simulink model "HL2"  (R2021b)
settings: Solver=FixedStepAuto  StartTime=0.0  StopTime=2  FixedStep=1/Fs  RelTol=1e-3
PreLoadFcn:
  | 50000
values from neighbouring files (symbols this model uses):
  Fs = 50000    [HL2.m]
libraries: fl_lib x208, ee_lib x58, nesl_utility x35
(part 1 of 3)
settings Model: Creator=fonzius  LastModifiedBy=fonzius

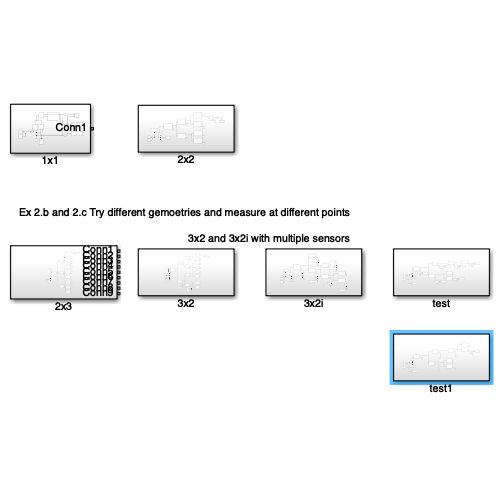
[thumbnail: Simulink's stored preview of the top-level diagram]
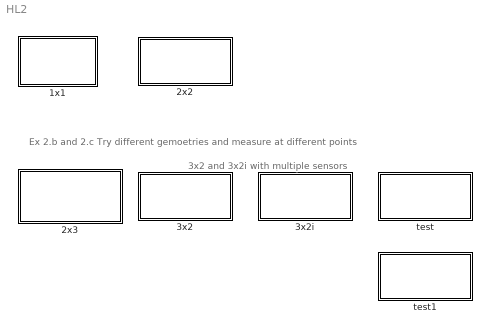
== system HL2 ==
  note: 3x2 and 3x2i with multiple sensors
  note: Ex 2.b and 2.c Try different gemoetries and measure at different points
  1x1 : Subsystem
  2x2 : Subsystem
  2x3 : Subsystem
  3x2 : Subsystem
  3x2i : Subsystem
  test : Subsystem
  test1 : Subsystem

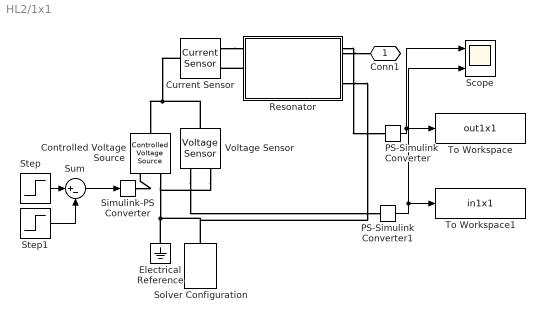
== system HL2/1x1 ==
  Controlled Voltage Source : fl_lib/Electrical/Electrical Sources/Controlled Voltage Source
  Current Sensor : fl_lib/Electrical/Electrical Sensors/Current Sensor
  Electrical Reference : fl_lib/Electrical/Electrical Elements/Electrical Reference
  PS-Simulink Converter : nesl_utility/PS-Simulink Converter  PhysicalDomain=network_engine_domain  SubClassName=ps_output  LeftPortType=input  RightPortType=output  PseudoPeriodic=off  Frequencies=[]  Unit=inherit  AffineConversion=off
      settings: SourceProductBaseCode=PW,SS
  PS-Simulink Converter1 : nesl_utility/PS-Simulink Converter  PhysicalDomain=network_engine_domain  SubClassName=ps_output  LeftPortType=input  RightPortType=output  PseudoPeriodic=off  Frequencies=[]  Unit=inherit  AffineConversion=off
      settings: SourceProductBaseCode=PW,SS
  Resonator : Subsystem
  Scope : Scope  NumInputPorts=2
  Simulink-PS Converter : nesl_utility/Simulink-PS Converter  PhysicalDomain=network_engine_domain  SubClassName=ps_input  LeftPortType=input  RightPortType=output  PseudoPeriodic=off  Frequencies=[]  NoiseDistribution=none  NoiseParameters=[]  Unit=1  AffineConversion=off  FilteringAndDerivatives=provide  SimscapeFilterOrder=1  InputFilterTimeConstant=0.001  UdotUserProvided=0
      settings: SourceProductBaseCode=PW,SS
  Solver Configuration : nesl_utility/Solver Configuration  PhysicalDomain=network_engine_domain  SubClassName=solver  LeftPortType=input  RightPortType=generic  Tones=[]  Harmonics=[]  SimulateNoise=off  Profile=off  UseLocalSampling=off  EnableSwitchedLinearOptims=on  FrequencyDomain=off  UseCCode=off  RelTol=0.001  AbsTol=1e-06  MinStep=1e-09  ToWorkspace=off  RevertToSquareIcSolve=off  NumHomotopyIterations=100  PhasorMode=off  PhasorModeNumHarmonics=1  DoDC=on  ResidualTolerance=1e-09  UseLocalSolver=off  LocalSolverChoice=NE_BACKWARD_EULER_ADVANCER  LocalSolverSampleTime=0.001  DoFixedCost=off  MaxNonlinIter=3  MaxModeIter=2  ComputeImpulses=off  ImpulseIterations=2  LinearAlgebra=auto  EquationFormulation=NE_TIME_EF  DelaysMemoryBudget=1024  AutomaticFiltering=on  FilteringTimeConstant=0.001  PartitionStorageMethod=AS_NEEDED  PartitionMemoryBudget=1024  PartitionMethod=ROBUST
      settings: SourceProductBaseCode=PW,SS
  Step : Step  Time=1/Fs  SampleTime=0
  Step1 : Step  Time=2/Fs  SampleTime=0
  Sum : Sum  Inputs=|+-
  To Workspace : ToWorkspace  VariableName=out1x1  SaveFormat=Timeseries  SampleTime=-1
  To Workspace1 : ToWorkspace  VariableName=in1x1  SaveFormat=Timeseries  SampleTime=-1
  Voltage Sensor : fl_lib/Electrical/Electrical Sensors/Voltage Sensor
  Conn1 : PMIOPort  Side=Right
  wires:
  Sum/1 -> Simulink-PS Converter/1
  PS-Simulink Converter/1 -> To Workspace/1, Scope/1
  Step/1 -> Sum/1
  PS-Simulink Converter1/1 -> Scope/2, To Workspace1/1
  Step1/1 -> Sum/2
  connections:
  Voltage Sensor/RConn1 -- PS-Simulink Converter1/LConn1
  Current Sensor/RConn1 -- PS-Simulink Converter/LConn1
  Electrical Reference/LConn1 -- Resonator/RConn2 -- Solver Configuration/RConn1 -- Voltage Sensor/RConn2 -- Controlled Voltage Source/RConn2
  Resonator/LConn1 -- Current Sensor/RConn2
  Simulink-PS Converter/RConn1 -- Controlled Voltage Source/RConn1
  Resonator/RConn1 -- Conn1/RConn1
  Voltage Sensor/LConn1 -- Current Sensor/LConn1 -- Controlled Voltage Source/LConn1

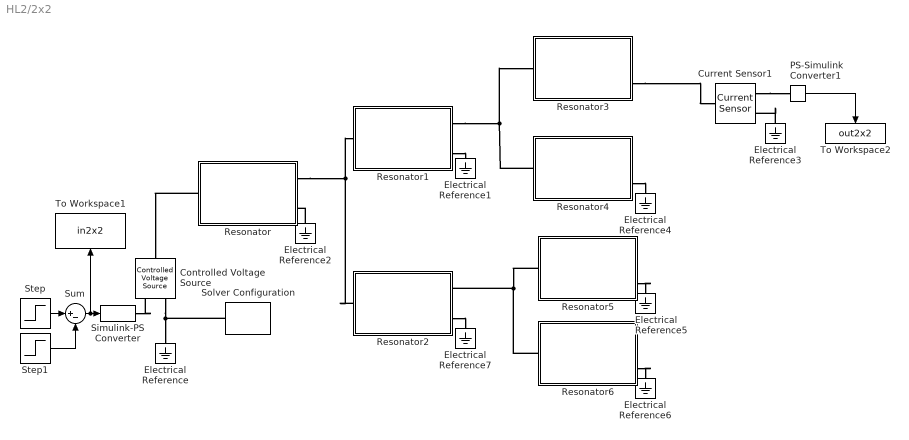
== system HL2/2x2 ==
  Controlled Voltage Source : fl_lib/Electrical/Electrical Sources/Controlled Voltage Source
  Current Sensor1 : fl_lib/Electrical/Electrical Sensors/Current Sensor
  Electrical Reference{,1..7} (8 alike) : fl_lib/Electrical/Electrical Elements/Electrical Reference
  PS-Simulink Converter1 : nesl_utility/PS-Simulink Converter  PhysicalDomain=network_engine_domain  SubClassName=ps_output  LeftPortType=input  RightPortType=output  PseudoPeriodic=off  Frequencies=[]  Unit=inherit  AffineConversion=off
      settings: SourceProductBaseCode=PW,SS
  Resonator : Subsystem
  Resonator1 : Subsystem
  Resonator2 : Subsystem
  Resonator3 : Subsystem
  Resonator4 : Subsystem
  Resonator5 : Subsystem
  Resonator6 : Subsystem
  Simulink-PS Converter : nesl_utility/Simulink-PS Converter  PhysicalDomain=network_engine_domain  SubClassName=ps_input  LeftPortType=input  RightPortType=output  PseudoPeriodic=off  Frequencies=[]  NoiseDistribution=none  NoiseParameters=[]  Unit=1  AffineConversion=off  FilteringAndDerivatives=provide  SimscapeFilterOrder=1  InputFilterTimeConstant=0.001  UdotUserProvided=0
      settings: SourceProductBaseCode=PW,SS
  Solver Configuration : nesl_utility/Solver Configuration  PhysicalDomain=network_engine_domain  SubClassName=solver  LeftPortType=input  RightPortType=generic  Tones=[]  Harmonics=[]  SimulateNoise=off  Profile=off  UseLocalSampling=off  EnableSwitchedLinearOptims=on  FrequencyDomain=off  UseCCode=off  RelTol=0.001  AbsTol=1e-06  MinStep=1e-09  ToWorkspace=off  RevertToSquareIcSolve=off  NumHomotopyIterations=100  PhasorMode=off  PhasorModeNumHarmonics=1  DoDC=on  ResidualTolerance=1e-09  UseLocalSolver=off  LocalSolverChoice=NE_BACKWARD_EULER_ADVANCER  LocalSolverSampleTime=0.001  DoFixedCost=off  MaxNonlinIter=3  MaxModeIter=2  ComputeImpulses=off  ImpulseIterations=2  LinearAlgebra=auto  EquationFormulation=NE_TIME_EF  DelaysMemoryBudget=1024  AutomaticFiltering=on  FilteringTimeConstant=0.001  PartitionStorageMethod=AS_NEEDED  PartitionMemoryBudget=1024  PartitionMethod=ROBUST
      settings: SourceProductBaseCode=PW,SS
  Step : Step  Time=1/Fs  SampleTime=0
  Step1 : Step  Time=2/Fs  SampleTime=0
  Sum : Sum  Inputs=|+-
  To Workspace1 : ToWorkspace  VariableName=in2x2  SaveFormat=Timeseries  SampleTime=-1
  To Workspace2 : ToWorkspace  VariableName=out2x2  SaveFormat=Timeseries  SampleTime=-1
  wires:
  Step1/1 -> Sum/2
  Step/1 -> Sum/1
  Sum/1 -> To Workspace1/1, Simulink-PS Converter/1
  PS-Simulink Converter1/1 -> To Workspace2/1
  connections:
  Resonator2/RConn2 -- Electrical Reference7/LConn1
  Resonator/RConn1 -- Resonator1/LConn1 -- Resonator2/LConn1
  Resonator5/RConn2 -- Electrical Reference5/LConn1
  Resonator4/RConn2 -- Electrical Reference4/LConn1
  Resonator1/RConn1 -- Resonator3/LConn1 -- Resonator4/LConn1
  Resonator5/LConn1 -- Resonator6/LConn1 -- Resonator2/RConn1
  Resonator6/RConn2 -- Electrical Reference6/LConn1
  Resonator/LConn1 -- Controlled Voltage Source/LConn1
  Simulink-PS Converter/RConn1 -- Controlled Voltage Source/RConn1
  Solver Configuration/RConn1 -- Electrical Reference/LConn1 -- Controlled Voltage Source/RConn2
  Current Sensor1/RConn1 -- PS-Simulink Converter1/LConn1
  Electrical Reference3/LConn1 -- Current Sensor1/RConn2
  Electrical Reference2/LConn1 -- Resonator/RConn2
  Resonator3/RConn2 -- Current Sensor1/LConn1
  Resonator1/RConn2 -- Electrical Reference1/LConn1

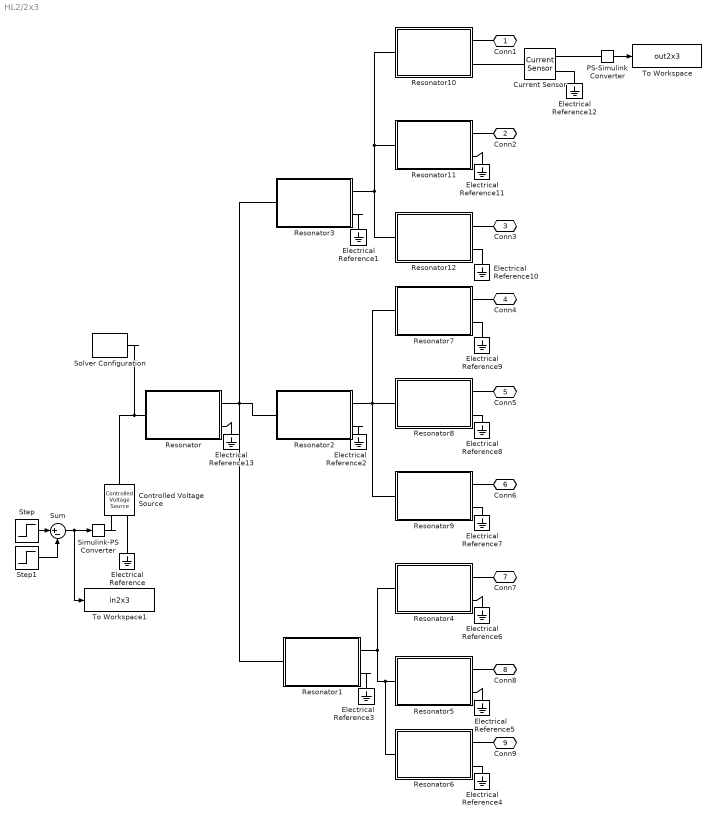
== system HL2/2x3 ==
  Controlled Voltage Source : fl_lib/Electrical/Electrical Sources/Controlled Voltage Source
  Current Sensor : fl_lib/Electrical/Electrical Sensors/Current Sensor
  Electrical Reference{,1..13} (14 alike) : fl_lib/Electrical/Electrical Elements/Electrical Reference
  PS-Simulink Converter : nesl_utility/PS-Simulink Converter  PhysicalDomain=network_engine_domain  SubClassName=ps_output  LeftPortType=input  RightPortType=output  PseudoPeriodic=off  Frequencies=[]  Unit=inherit  AffineConversion=off
      settings: SourceProductBaseCode=PW,SS
  Resonator : Subsystem
  Resonator1 : Subsystem
  Resonator10 : Subsystem
  Resonator11 : Subsystem
  Resonator12 : Subsystem
  Resonator2 : Subsystem
  Resonator3 : Subsystem
  Resonator4 : Subsystem
  Resonator5 : Subsystem
  Resonator6 : Subsystem
  Resonator7 : Subsystem
  Resonator8 : Subsystem
  Resonator9 : Subsystem
  Simulink-PS Converter : nesl_utility/Simulink-PS Converter  PhysicalDomain=network_engine_domain  SubClassName=ps_input  LeftPortType=input  RightPortType=output  PseudoPeriodic=off  Frequencies=[]  NoiseDistribution=none  NoiseParameters=[]  Unit=1  AffineConversion=off  FilteringAndDerivatives=provide  SimscapeFilterOrder=1  InputFilterTimeConstant=0.001  UdotUserProvided=0
      settings: SourceProductBaseCode=PW,SS
  Solver Configuration : nesl_utility/Solver Configuration  PhysicalDomain=network_engine_domain  SubClassName=solver  LeftPortType=input  RightPortType=generic  Tones=[]  Harmonics=[]  SimulateNoise=off  Profile=off  UseLocalSampling=off  EnableSwitchedLinearOptims=on  FrequencyDomain=off  UseCCode=off  RelTol=0.001  AbsTol=1e-06  MinStep=1e-09  ToWorkspace=off  RevertToSquareIcSolve=off  NumHomotopyIterations=100  PhasorMode=off  PhasorModeNumHarmonics=1  DoDC=on  ResidualTolerance=1e-09  UseLocalSolver=off  LocalSolverChoice=NE_BACKWARD_EULER_ADVANCER  LocalSolverSampleTime=0.001  DoFixedCost=off  MaxNonlinIter=3  MaxModeIter=2  ComputeImpulses=off  ImpulseIterations=2  LinearAlgebra=auto  EquationFormulation=NE_TIME_EF  DelaysMemoryBudget=1024  AutomaticFiltering=on  FilteringTimeConstant=0.001  PartitionStorageMethod=AS_NEEDED  PartitionMemoryBudget=1024  PartitionMethod=ROBUST
      settings: SourceProductBaseCode=PW,SS
  Step : Step  Time=1/Fs  SampleTime=0
  Step1 : Step  Time=2/Fs  SampleTime=0
  Sum : Sum  Inputs=|+-
  To Workspace : ToWorkspace  VariableName=out2x3  SaveFormat=Timeseries  SampleTime=-1
  To Workspace1 : ToWorkspace  VariableName=in2x3  SaveFormat=Timeseries  SampleTime=-1
  Conn1 : PMIOPort  Side=Right
  Conn2 : PMIOPort  Port=2  Side=Right
  Conn3 : PMIOPort  Port=3  Side=Right
  Conn4 : PMIOPort  Port=4  Side=Right
  Conn5 : PMIOPort  Port=5  Side=Right
  Conn6 : PMIOPort  Port=6  Side=Right
  Conn7 : PMIOPort  Port=7  Side=Right
  Conn8 : PMIOPort  Port=8  Side=Right
  Conn9 : PMIOPort  Port=9  Side=Right
  wires:
  Step/1 -> Sum/1
  Sum/1 -> To Workspace1/1, Simulink-PS Converter/1
  Step1/1 -> Sum/2
  PS-Simulink Converter/1 -> To Workspace/1
  connections:
  Resonator9/RConn1 -- Conn6/RConn1
  Resonator11/RConn1 -- Conn2/RConn1
  Resonator12/RConn1 -- Conn3/RConn1
  Resonator7/RConn2 -- Electrical Reference9/LConn1
  Resonator1/RConn2 -- Electrical Reference3/LConn1
  Resonator9/RConn2 -- Electrical Reference7/LConn1
  Resonator3/RConn2 -- Electrical Reference1/LConn1
  Resonator2/RConn2 -- Electrical Reference2/LConn1
  Simulink-PS Converter/RConn1 -- Controlled Voltage Source/RConn1
  Resonator6/RConn1 -- Conn9/RConn1
  Resonator4/RConn1 -- Conn7/RConn1
  Electrical Reference11/LConn1 -- Resonator11/RConn2
  Resonator4/LConn1 -- Resonator6/LConn1 -- Resonator5/LConn1 -- Resonator1/RConn1
  Resonator/RConn1 -- Resonator1/LConn1 -- Resonator3/LConn1 -- Resonator2/LConn1
  Electrical Reference5/LConn1 -- Resonator5/RConn2
  Resonator7/RConn1 -- Conn4/RConn1
  Resonator10/RConn2 -- Current Sensor/LConn1
  Solver Configuration/RConn1 -- Controlled Voltage Source/LConn1 -- Resonator/LConn1
  Resonator2/RConn1 -- Resonator8/LConn1 -- Resonator9/LConn1 -- Resonator7/LConn1
  Resonator8/RConn1 -- Conn5/RConn1
  Resonator8/RConn2 -- Electrical Reference8/LConn1
  Resonator10/LConn1 -- Resonator11/LConn1 -- Resonator12/LConn1 -- Resonator3/RConn1
  Resonator12/RConn2 -- Electrical Reference10/LConn1
  Resonator10/RConn1 -- Conn1/RConn1
  Resonator6/RConn2 -- Electrical Reference4/LConn1
  Electrical Reference13/LConn1 -- Resonator/RConn2
  Resonator5/RConn1 -- Conn8/RConn1
  Electrical Reference6/LConn1 -- Resonator4/RConn2
  Controlled Voltage Source/RConn2 -- Electrical Reference/LConn1
  Current Sensor/RConn1 -- PS-Simulink Converter/LConn1
  Electrical Reference12/LConn1 -- Current Sensor/RConn2

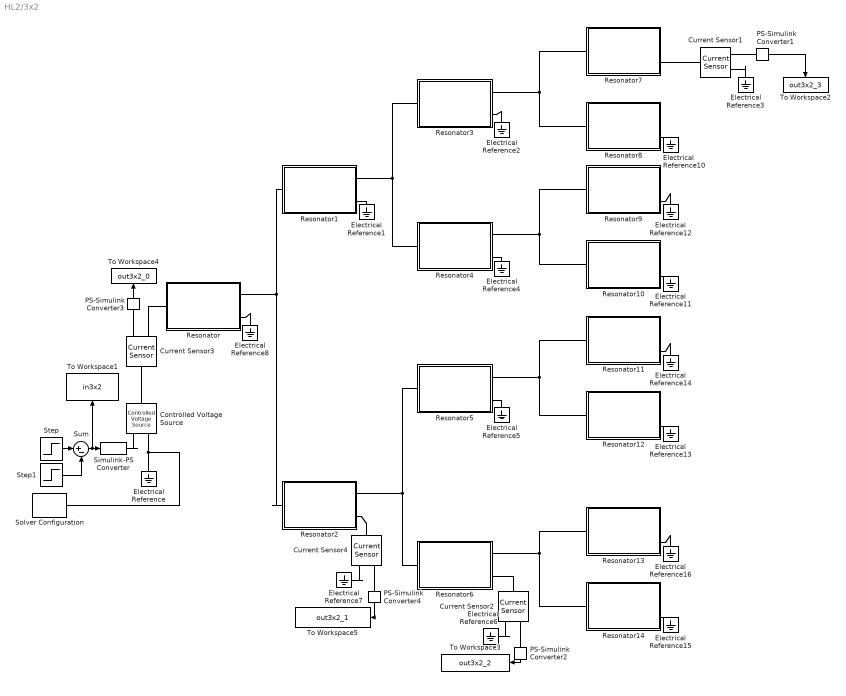
== system HL2/3x2 ==
  Controlled Voltage Source : fl_lib/Electrical/Electrical Sources/Controlled Voltage Source
  Current Sensor{1..4} (4 alike) : fl_lib/Electrical/Electrical Sensors/Current Sensor
  Electrical Reference{,1..8,10..16} (16 alike) : fl_lib/Electrical/Electrical Elements/Electrical Reference
  PS-Simulink Converter{1..4} (4 alike) : nesl_utility/PS-Simulink Converter  PhysicalDomain=network_engine_domain  SubClassName=ps_output  LeftPortType=input  RightPortType=output  PseudoPeriodic=off  Frequencies=[]  Unit=inherit  AffineConversion=off
      settings: SourceProductBaseCode=PW,SS
  Resonator : Subsystem
  Resonator1 : Subsystem
  Resonator10 : Subsystem
  Resonator11 : Subsystem
  Resonator12 : Subsystem
  Resonator13 : Subsystem
  Resonator14 : Subsystem
  Resonator2 : Subsystem
  Resonator3 : Subsystem
  Resonator4 : Subsystem
  Resonator5 : Subsystem
  Resonator6 : Subsystem
  Resonator7 : Subsystem
  Resonator8 : Subsystem
  Resonator9 : Subsystem
  Simulink-PS Converter : nesl_utility/Simulink-PS Converter  PhysicalDomain=network_engine_domain  SubClassName=ps_input  LeftPortType=input  RightPortType=output  PseudoPeriodic=off  Frequencies=[]  NoiseDistribution=none  NoiseParameters=[]  Unit=1  AffineConversion=off  FilteringAndDerivatives=provide  SimscapeFilterOrder=1  InputFilterTimeConstant=0.001  UdotUserProvided=0
      settings: SourceProductBaseCode=PW,SS
  Solver Configuration : nesl_utility/Solver Configuration  PhysicalDomain=network_engine_domain  SubClassName=solver  LeftPortType=input  RightPortType=generic  Tones=[]  Harmonics=[]  SimulateNoise=off  Profile=off  UseLocalSampling=off  EnableSwitchedLinearOptims=on  FrequencyDomain=off  UseCCode=off  RelTol=0.001  AbsTol=1e-06  MinStep=1e-09  ToWorkspace=off  RevertToSquareIcSolve=off  NumHomotopyIterations=100  PhasorMode=off  PhasorModeNumHarmonics=1  DoDC=on  ResidualTolerance=1e-09  UseLocalSolver=off  LocalSolverChoice=NE_BACKWARD_EULER_ADVANCER  LocalSolverSampleTime=0.001  DoFixedCost=off  MaxNonlinIter=3  MaxModeIter=2  ComputeImpulses=off  ImpulseIterations=2  LinearAlgebra=auto  EquationFormulation=NE_TIME_EF  DelaysMemoryBudget=1024  AutomaticFiltering=on  FilteringTimeConstant=0.001  PartitionStorageMethod=AS_NEEDED  PartitionMemoryBudget=1024  PartitionMethod=ROBUST
      settings: SourceProductBaseCode=PW,SS
  Step : Step  Time=1/Fs  SampleTime=0
  Step1 : Step  Time=2/Fs  SampleTime=0
  Sum : Sum  Inputs=|+-
  To Workspace1 : ToWorkspace  VariableName=in3x2  SaveFormat=Timeseries  SampleTime=-1
  To Workspace2 : ToWorkspace  VariableName=out3x2_3  SaveFormat=Timeseries  SampleTime=-1
  To Workspace3 : ToWorkspace  VariableName=out3x2_2  SaveFormat=Timeseries  SampleTime=-1
  To Workspace4 : ToWorkspace  VariableName=out3x2_0  SaveFormat=Timeseries  SampleTime=-1
  To Workspace5 : ToWorkspace  VariableName=out3x2_1  SaveFormat=Timeseries  SampleTime=-1
  wires:
  Step1/1 -> Sum/2
  Step/1 -> Sum/1
  Sum/1 -> To Workspace1/1, Simulink-PS Converter/1
  PS-Simulink Converter3/1 -> To Workspace4/1
  PS-Simulink Converter1/1 -> To Workspace2/1
  PS-Simulink Converter2/1 -> To Workspace3/1
  PS-Simulink Converter4/1 -> To Workspace5/1
  connections:
  Current Sensor4/LConn1 -- Resonator2/RConn2
  Resonator/RConn1 -- Resonator1/LConn1 -- Resonator2/LConn1
  Resonator5/RConn2 -- Electrical Reference5/LConn1
  Resonator4/RConn2 -- Electrical Reference4/LConn1
  Resonator1/RConn1 -- Resonator4/LConn1 -- Resonator3/LConn1
  Resonator5/LConn1 -- Resonator6/LConn1 -- Resonator2/RConn1
  Current Sensor2/LConn1 -- Resonator6/RConn2
  Simulink-PS Converter/RConn1 -- Controlled Voltage Source/RConn1
  Solver Configuration/RConn1 -- Electrical Reference/LConn1 -- Controlled Voltage Source/RConn2
  Current Sensor3/RConn1 -- PS-Simulink Converter3/LConn1
  Resonator1/RConn2 -- Electrical Reference1/LConn1
  Electrical Reference3/LConn1 -- Current Sensor1/RConn2
  Current Sensor1/RConn1 -- PS-Simulink Converter1/LConn1
  Electrical Reference2/LConn1 -- Resonator3/RConn2
  Resonator8/RConn2 -- Electrical Reference10/LConn1
  Resonator7/RConn2 -- Current Sensor1/LConn1
  Resonator7/LConn1 -- Resonator8/LConn1 -- Resonator3/RConn1
  Electrical Reference12/LConn1 -- Resonator9/RConn2
  Resonator10/RConn2 -- Electrical Reference11/LConn1
  Resonator9/LConn1 -- Resonator10/LConn1 -- Resonator4/RConn1
  Electrical Reference14/LConn1 -- Resonator11/RConn2
  Resonator12/RConn2 -- Electrical Reference13/LConn1
  Resonator11/LConn1 -- Resonator12/LConn1 -- Resonator5/RConn1
  Electrical Reference16/LConn1 -- Resonator13/RConn2
  Resonator14/RConn2 -- Electrical Reference15/LConn1
  Resonator6/RConn1 -- Resonator14/LConn1 -- Resonator13/LConn1
  Electrical Reference8/LConn1 -- Resonator/RConn2
  Current Sensor3/LConn1 -- Controlled Voltage Source/LConn1
  Resonator/LConn1 -- Current Sensor3/RConn2
  Current Sensor2/RConn1 -- PS-Simulink Converter2/LConn1
  Electrical Reference6/LConn1 -- Current Sensor2/RConn2
  Electrical Reference7/LConn1 -- Current Sensor4/RConn2
  Current Sensor4/RConn1 -- PS-Simulink Converter4/LConn1

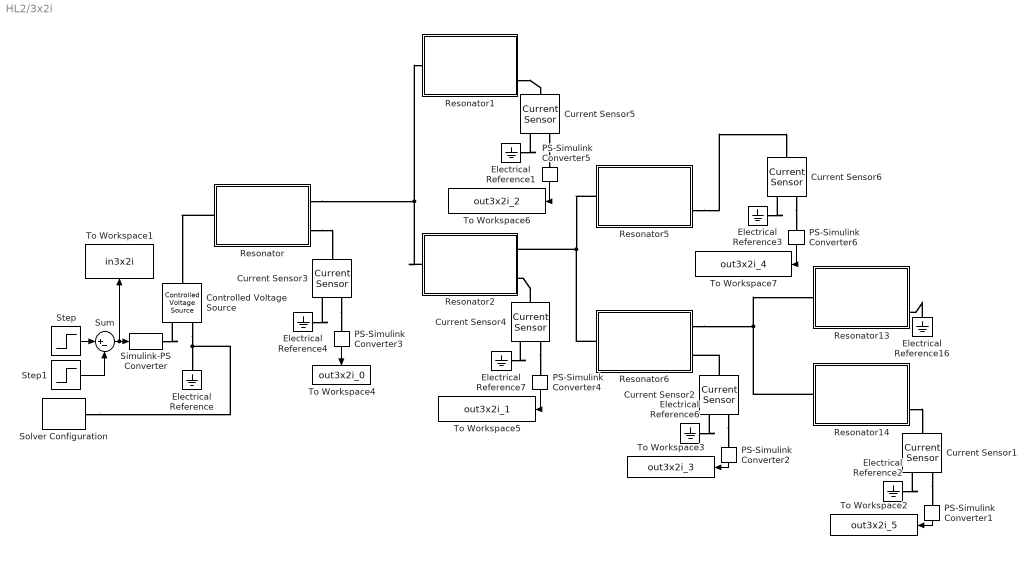
== system HL2/3x2i ==
  Controlled Voltage Source : fl_lib/Electrical/Electrical Sources/Controlled Voltage Source
  Current Sensor{1..6} (6 alike) : fl_lib/Electrical/Electrical Sensors/Current Sensor
  Electrical Reference{,1..4,6..7,16} (8 alike) : fl_lib/Electrical/Electrical Elements/Electrical Reference
  PS-Simulink Converter{1..6} (6 alike) : nesl_utility/PS-Simulink Converter  PhysicalDomain=network_engine_domain  SubClassName=ps_output  LeftPortType=input  RightPortType=output  PseudoPeriodic=off  Frequencies=[]  Unit=inherit  AffineConversion=off
      settings: SourceProductBaseCode=PW,SS
  Resonator : Subsystem
  Resonator1 : Subsystem
  Resonator13 : Subsystem
  Resonator14 : Subsystem
  Resonator2 : Subsystem
  Resonator5 : Subsystem
  Resonator6 : Subsystem
  Simulink-PS Converter : nesl_utility/Simulink-PS Converter  PhysicalDomain=network_engine_domain  SubClassName=ps_input  LeftPortType=input  RightPortType=output  PseudoPeriodic=off  Frequencies=[]  NoiseDistribution=none  NoiseParameters=[]  Unit=1  AffineConversion=off  FilteringAndDerivatives=provide  SimscapeFilterOrder=1  InputFilterTimeConstant=0.001  UdotUserProvided=0
      settings: SourceProductBaseCode=PW,SS
  Solver Configuration : nesl_utility/Solver Configuration  PhysicalDomain=network_engine_domain  SubClassName=solver  LeftPortType=input  RightPortType=generic  Tones=[]  Harmonics=[]  SimulateNoise=off  Profile=off  UseLocalSampling=off  EnableSwitchedLinearOptims=on  FrequencyDomain=off  UseCCode=off  RelTol=0.001  AbsTol=1e-06  MinStep=1e-09  ToWorkspace=off  RevertToSquareIcSolve=off  NumHomotopyIterations=100  PhasorMode=off  PhasorModeNumHarmonics=1  DoDC=on  ResidualTolerance=1e-09  UseLocalSolver=off  LocalSolverChoice=NE_BACKWARD_EULER_ADVANCER  LocalSolverSampleTime=0.001  DoFixedCost=off  MaxNonlinIter=3  MaxModeIter=2  ComputeImpulses=off  ImpulseIterations=2  LinearAlgebra=auto  EquationFormulation=NE_TIME_EF  DelaysMemoryBudget=1024  AutomaticFiltering=on  FilteringTimeConstant=0.001  PartitionStorageMethod=AS_NEEDED  PartitionMemoryBudget=1024  PartitionMethod=ROBUST
      settings: SourceProductBaseCode=PW,SS
  Step : Step  Time=1/Fs  SampleTime=0
  Step1 : Step  Time=2/Fs  SampleTime=0
  Sum : Sum  Inputs=|+-
  To Workspace1 : ToWorkspace  VariableName=in3x2i  SaveFormat=Timeseries  SampleTime=-1
  To Workspace2 : ToWorkspace  VariableName=out3x2i_5  SaveFormat=Timeseries  SampleTime=-1
  To Workspace3 : ToWorkspace  VariableName=out3x2i_3  SaveFormat=Timeseries  SampleTime=-1
  To Workspace4 : ToWorkspace  VariableName=out3x2i_0  SaveFormat=Timeseries  SampleTime=-1
  To Workspace5 : ToWorkspace  VariableName=out3x2i_1  SaveFormat=Timeseries  SampleTime=-1
  To Workspace6 : ToWorkspace  VariableName=out3x2i_2  SaveFormat=Timeseries  SampleTime=-1
  To Workspace7 : ToWorkspace  VariableName=out3x2i_4  SaveFormat=Timeseries  SampleTime=-1
  wires:
  Step1/1 -> Sum/2
  Step/1 -> Sum/1
  Sum/1 -> To Workspace1/1, Simulink-PS Converter/1
  PS-Simulink Converter2/1 -> To Workspace3/1
  PS-Simulink Converter4/1 -> To Workspace5/1
  PS-Simulink Converter1/1 -> To Workspace2/1
  PS-Simulink Converter5/1 -> To Workspace6/1
  PS-Simulink Converter6/1 -> To Workspace7/1
  PS-Simulink Converter3/1 -> To Workspace4/1
  connections:
  Current Sensor4/LConn1 -- Resonator2/RConn2
  Resonator/RConn1 -- Resonator1/LConn1 -- Resonator2/LConn1
  Resonator5/RConn2 -- Current Sensor6/LConn1
  Resonator5/LConn1 -- Resonator6/LConn1 -- Resonator2/RConn1
  Current Sensor2/LConn1 -- Resonator6/RConn2
  Simulink-PS Converter/RConn1 -- Controlled Voltage Source/RConn1
  Solver Configuration/RConn1 -- Electrical Reference/LConn1 -- Controlled Voltage Source/RConn2
  Resonator1/RConn2 -- Current Sensor5/LConn1
  Electrical Reference16/LConn1 -- Resonator13/RConn2
  Resonator14/RConn2 -- Current Sensor1/LConn1
  Resonator6/RConn1 -- Resonator13/LConn1 -- Resonator14/LConn1
  Resonator/LConn1 -- Controlled Voltage Source/LConn1
  Current Sensor2/RConn1 -- PS-Simulink Converter2/LConn1
  Electrical Reference6/LConn1 -- Current Sensor2/RConn2
  Electrical Reference7/LConn1 -- Current Sensor4/RConn2
  Current Sensor4/RConn1 -- PS-Simulink Converter4/LConn1
  Current Sensor1/RConn1 -- PS-Simulink Converter1/LConn1
  Electrical Reference2/LConn1 -- Current Sensor1/RConn2
  Electrical Reference1/LConn1 -- Current Sensor5/RConn2
  Current Sensor5/RConn1 -- PS-Simulink Converter5/LConn1
  Electrical Reference3/LConn1 -- Current Sensor6/RConn2
  Current Sensor6/RConn1 -- PS-Simulink Converter6/LConn1
  Current Sensor3/RConn1 -- PS-Simulink Converter3/LConn1
  Electrical Reference4/LConn1 -- Current Sensor3/RConn2
  Resonator/RConn2 -- Current Sensor3/LConn1

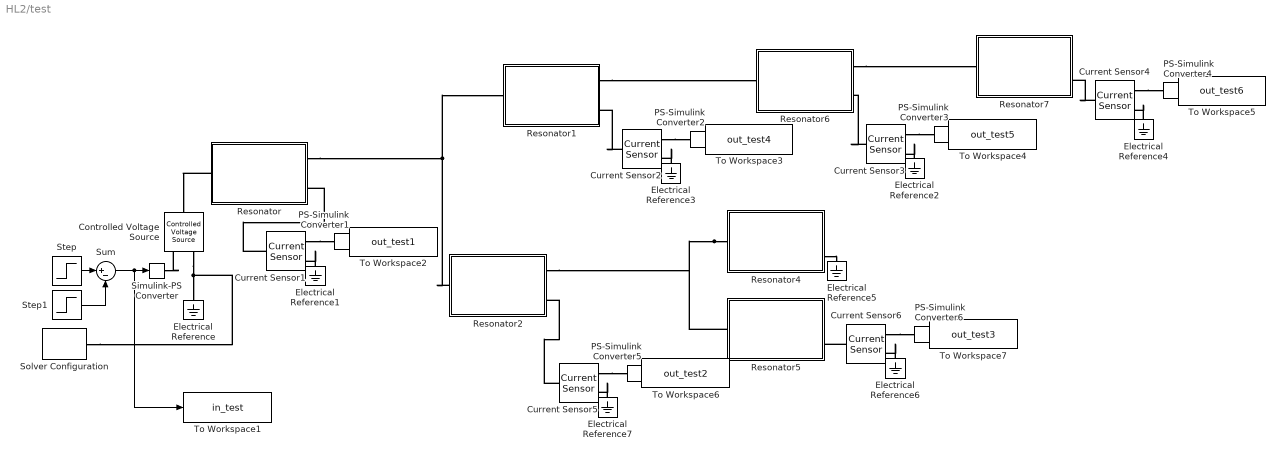
== system HL2/test ==
  Controlled Voltage Source : fl_lib/Electrical/Electrical Sources/Controlled Voltage Source
  Current Sensor{1..6} (6 alike) : fl_lib/Electrical/Electrical Sensors/Current Sensor
  Electrical Reference{,1..7} (8 alike) : fl_lib/Electrical/Electrical Elements/Electrical Reference
  PS-Simulink Converter{1..6} (6 alike) : nesl_utility/PS-Simulink Converter  PhysicalDomain=network_engine_domain  SubClassName=ps_output  LeftPortType=input  RightPortType=output  PseudoPeriodic=off  Frequencies=[]  Unit=inherit  AffineConversion=off
      settings: SourceProductBaseCode=PW,SS
  Resonator : Subsystem
  Resonator1 : Subsystem
  Resonator2 : Subsystem
  Resonator4 : Subsystem
  Resonator5 : Subsystem
  Resonator6 : Subsystem
  Resonator7 : Subsystem
  Simulink-PS Converter : nesl_utility/Simulink-PS Converter  PhysicalDomain=network_engine_domain  SubClassName=ps_input  LeftPortType=input  RightPortType=output  PseudoPeriodic=off  Frequencies=[]  NoiseDistribution=none  NoiseParameters=[]  Unit=1  AffineConversion=off  FilteringAndDerivatives=provide  SimscapeFilterOrder=1  InputFilterTimeConstant=0.001  UdotUserProvided=0
      settings: SourceProductBaseCode=PW,SS
  Solver Configuration : nesl_utility/Solver Configuration  PhysicalDomain=network_engine_domain  SubClassName=solver  LeftPortType=input  RightPortType=generic  Tones=[]  Harmonics=[]  SimulateNoise=off  Profile=off  UseLocalSampling=off  EnableSwitchedLinearOptims=on  FrequencyDomain=off  UseCCode=off  RelTol=0.001  AbsTol=1e-06  MinStep=1e-09  ToWorkspace=off  RevertToSquareIcSolve=off  NumHomotopyIterations=100  PhasorMode=off  PhasorModeNumHarmonics=1  DoDC=on  ResidualTolerance=1e-09  UseLocalSolver=off  LocalSolverChoice=NE_BACKWARD_EULER_ADVANCER  LocalSolverSampleTime=0.001  DoFixedCost=off  MaxNonlinIter=3  MaxModeIter=2  ComputeImpulses=off  ImpulseIterations=2  LinearAlgebra=auto  EquationFormulation=NE_TIME_EF  DelaysMemoryBudget=1024  AutomaticFiltering=on  FilteringTimeConstant=0.001  PartitionStorageMethod=AS_NEEDED  PartitionMemoryBudget=1024  PartitionMethod=ROBUST
      settings: SourceProductBaseCode=PW,SS
  Step : Step  Time=1/Fs  SampleTime=0
  Step1 : Step  Time=2/Fs  SampleTime=0
  Sum : Sum  Inputs=|+-
  To Workspace1 : ToWorkspace  VariableName=in_test  SaveFormat=Timeseries  SampleTime=-1
  To Workspace2 : ToWorkspace  VariableName=out_test1  SaveFormat=Timeseries  SampleTime=-1
  To Workspace3 : ToWorkspace  VariableName=out_test4  SaveFormat=Timeseries  SampleTime=-1
  To Workspace4 : ToWorkspace  VariableName=out_test5  SaveFormat=Timeseries  SampleTime=-1
  To Workspace5 : ToWorkspace  VariableName=out_test6  SaveFormat=Timeseries  SampleTime=-1
  To Workspace6 : ToWorkspace  VariableName=out_test2  SaveFormat=Timeseries  SampleTime=-1
  To Workspace7 : ToWorkspace  VariableName=out_test3  SaveFormat=Timeseries  SampleTime=-1
  wires:
  Step/1 -> Sum/1
  Step1/1 -> Sum/2
  Sum/1 -> To Workspace1/1, Simulink-PS Converter/1
  PS-Simulink Converter2/1 -> To Workspace3/1
  PS-Simulink Converter3/1 -> To Workspace4/1
  PS-Simulink Converter4/1 -> To Workspace5/1
  PS-Simulink Converter5/1 -> To Workspace6/1
  PS-Simulink Converter6/1 -> To Workspace7/1
  PS-Simulink Converter1/1 -> To Workspace2/1
  connections:
  Resonator2/LConn1 -- Resonator/RConn1 -- Resonator1/LConn1
  Resonator4/LConn1 -- Resonator2/RConn1 -- Resonator5/LConn1
  Controlled Voltage Source/RConn2 -- Solver Configuration/RConn1 -- Electrical Reference/LConn1
  Current Sensor6/LConn1 -- Resonator5/RConn2
  Current Sensor3/LConn1 -- Resonator6/RConn2
  Resonator/LConn1 -- Controlled Voltage Source/LConn1
  Current Sensor5/LConn1 -- Resonator2/RConn2
  Current Sensor2/LConn1 -- Resonator1/RConn2
  Resonator4/RConn2 -- Electrical Reference5/LConn1
  Current Sensor4/LConn1 -- Resonator7/RConn2
  Simulink-PS Converter/RConn1 -- Controlled Voltage Source/RConn1
  Resonator1/RConn1 -- Resonator6/LConn1
  Resonator6/RConn1 -- Resonator7/LConn1
  Electrical Reference3/LConn1 -- Current Sensor2/RConn2
  Current Sensor2/RConn1 -- PS-Simulink Converter2/LConn1
  Electrical Reference2/LConn1 -- Current Sensor3/RConn2
  Current Sensor3/RConn1 -- PS-Simulink Converter3/LConn1
  Electrical Reference4/LConn1 -- Current Sensor4/RConn2
  Current Sensor4/RConn1 -- PS-Simulink Converter4/LConn1
  Electrical Reference7/LConn1 -- Current Sensor5/RConn2
  Current Sensor5/RConn1 -- PS-Simulink Converter5/LConn1
  Electrical Reference6/LConn1 -- Current Sensor6/RConn2
  Current Sensor6/RConn1 -- PS-Simulink Converter6/LConn1
  Electrical Reference1/LConn1 -- Current Sensor1/RConn2
  Current Sensor1/RConn1 -- PS-Simulink Converter1/LConn1
  Current Sensor1/LConn1 -- Resonator/RConn2

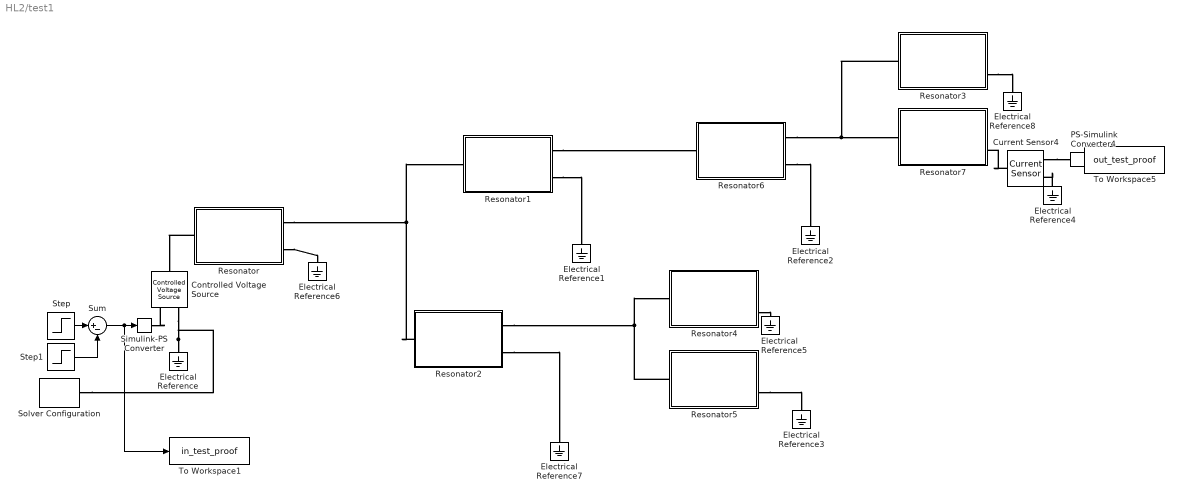
== system HL2/test1 ==
  Controlled Voltage Source : fl_lib/Electrical/Electrical Sources/Controlled Voltage Source
  Current Sensor4 : fl_lib/Electrical/Electrical Sensors/Current Sensor
  Electrical Reference{,1..8} (9 alike) : fl_lib/Electrical/Electrical Elements/Electrical Reference
  PS-Simulink Converter4 : nesl_utility/PS-Simulink Converter  PhysicalDomain=network_engine_domain  SubClassName=ps_output  LeftPortType=input  RightPortType=output  PseudoPeriodic=off  Frequencies=[]  Unit=inherit  AffineConversion=off
      settings: SourceProductBaseCode=PW,SS
  Resonator : Subsystem
  Resonator1 : Subsystem
  Resonator2 : Subsystem
  Resonator3 : Subsystem
  Resonator4 : Subsystem
  Resonator5 : Subsystem
  Resonator6 : Subsystem
  Resonator7 : Subsystem
  Simulink-PS Converter : nesl_utility/Simulink-PS Converter  PhysicalDomain=network_engine_domain  SubClassName=ps_input  LeftPortType=input  RightPortType=output  PseudoPeriodic=off  Frequencies=[]  NoiseDistribution=none  NoiseParameters=[]  Unit=1  AffineConversion=off  FilteringAndDerivatives=provide  SimscapeFilterOrder=1  InputFilterTimeConstant=0.001  UdotUserProvided=0
      settings: SourceProductBaseCode=PW,SS
  Solver Configuration : nesl_utility/Solver Configuration  PhysicalDomain=network_engine_domain  SubClassName=solver  LeftPortType=input  RightPortType=generic  Tones=[]  Harmonics=[]  SimulateNoise=off  Profile=off  UseLocalSampling=off  EnableSwitchedLinearOptims=on  FrequencyDomain=off  UseCCode=off  RelTol=0.001  AbsTol=1e-06  MinStep=1e-09  ToWorkspace=off  RevertToSquareIcSolve=off  NumHomotopyIterations=100  PhasorMode=off  PhasorModeNumHarmonics=1  DoDC=on  ResidualTolerance=1e-09  UseLocalSolver=off  LocalSolverChoice=NE_BACKWARD_EULER_ADVANCER  LocalSolverSampleTime=0.001  DoFixedCost=off  MaxNonlinIter=3  MaxModeIter=2  ComputeImpulses=off  ImpulseIterations=2  LinearAlgebra=auto  EquationFormulation=NE_TIME_EF  DelaysMemoryBudget=1024  AutomaticFiltering=on  FilteringTimeConstant=0.001  PartitionStorageMethod=AS_NEEDED  PartitionMemoryBudget=1024  PartitionMethod=ROBUST
      settings: SourceProductBaseCode=PW,SS
  Step : Step  Time=1/Fs  SampleTime=0
  Step1 : Step  Time=2/Fs  SampleTime=0
  Sum : Sum  Inputs=|+-
  To Workspace1 : ToWorkspace  VariableName=in_test_proof  SaveFormat=Timeseries  SampleTime=-1
  To Workspace5 : ToWorkspace  VariableName=out_test_proof  SaveFormat=Timeseries  SampleTime=-1
  wires:
  Step/1 -> Sum/1
  Step1/1 -> Sum/2
  Sum/1 -> To Workspace1/1, Simulink-PS Converter/1
  PS-Simulink Converter4/1 -> To Workspace5/1
  connections:
  Resonator2/LConn1 -- Resonator1/LConn1 -- Resonator/RConn1
  Resonator5/LConn1 -- Resonator4/LConn1 -- Resonator2/RConn1
  Electrical Reference/LConn1 -- Controlled Voltage Source/RConn2 -- Solver Configuration/RConn1
  Resonator5/RConn2 -- Electrical Reference3/LConn1
  Resonator6/RConn2 -- Electrical Reference2/LConn1
  Resonator/LConn1 -- Controlled Voltage Source/LConn1
  Resonator1/RConn2 -- Electrical Reference1/LConn1
  Resonator4/RConn2 -- Electrical Reference5/LConn1
  Current Sensor4/LConn1 -- Resonator7/RConn2
  Simulink-PS Converter/RConn1 -- Controlled Voltage Source/RConn1
  Resonator1/RConn1 -- Resonator6/LConn1
  Resonator6/RConn1 -- Resonator3/LConn1 -- Resonator7/LConn1
  Electrical Reference4/LConn1 -- Current Sensor4/RConn2
  Current Sensor4/RConn1 -- PS-Simulink Converter4/LConn1
  Resonator2/RConn2 -- Electrical Reference7/LConn1
  Resonator/RConn2 -- Electrical Reference6/LConn1
  Resonator3/RConn2 -- Electrical Reference8/LConn1

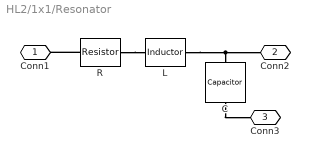
== system HL2/1x1/Resonator ==
  C : fl_lib/Electrical/Electrical Elements/Capacitor  c=7.0832e-07 F  r=0 Ohm  g=0 1/Ohm  i_specify=off  i_priority=None  i=0 A  i_nominal_specify=off  i_nominal_unit=A  i_nominal_value=1  v_specify=off  v_priority=None  v=0 V  v_nominal_specify=off  v_nominal_unit=V  v_nominal_value=1  vc_specify=off  vc_priority=High  vc=0 V  vc_nominal_specify=off  vc_nominal_unit=V  vc_nominal_value=1
  L : ee_lib/Passive/Inductor  l=0.10005 H  L_tol=0  enable_L_tol=0  tol_distribution=1  nSigma=4  r=0 Ohm  g=0 1/Ohm  enable_operating_limits=0  operating_limit_action=2  max_working_current=1 A  power_rating=1 W  enable_faults=0  fault_action=1  lambdaPercent=50  k_faulted=0.9999  turnsShort=0  openCct=0  groundShort=0  groundShortG=0 1/Ohm  tau_fault=1e-3 s  enable_temporal_fault=0  t_fault=1 s  enable_behavioral_fault=0  max_permissible_voltage=100 V  n_fail_on_voltage=1  max_permissible_current=1 A  t_fail_on_current=1 s  i_L_specify=off  i_L_priority=High  i_L=0 A  i_L_nominal_specify=off  i_L_nominal_unit=A  i_L_nominal_value=1
  R : fl_lib/Electrical/Electrical Elements/Resistor  R=4.116 Ohm  i_specify=off  i_priority=None  i=0 A  i_nominal_specify=off  i_nominal_unit=A  i_nominal_value=1  v_specify=off  v_priority=None  v=0 V  v_nominal_specify=off  v_nominal_unit=V  v_nominal_value=1
  Conn1 : PMIOPort  Side=Left
  Conn2 : PMIOPort  Port=2  Side=Right
  Conn3 : PMIOPort  Port=3  Side=Right
  connections:
  R/RConn1 -- L/LConn1
  C/RConn1 -- Conn3/RConn1
  R/LConn1 -- Conn1/RConn1
  L/RConn1 -- Conn2/RConn1 -- C/LConn1

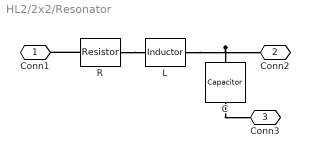
== system HL2/2x2/Resonator ==
  C : fl_lib/Electrical/Electrical Elements/Capacitor  c=7.0832e-07 F  r=0 Ohm  g=0 1/Ohm  i_specify=off  i_priority=None  i=0 A  i_nominal_specify=off  i_nominal_unit=A  i_nominal_value=1  v_specify=off  v_priority=None  v=0 V  v_nominal_specify=off  v_nominal_unit=V  v_nominal_value=1  vc_specify=off  vc_priority=High  vc=0 V  vc_nominal_specify=off  vc_nominal_unit=V  vc_nominal_value=1
  L : ee_lib/Passive/Inductor  l=0.10005 H  L_tol=0  enable_L_tol=0  tol_distribution=1  nSigma=4  r=0 Ohm  g=0 1/Ohm  enable_operating_limits=0  operating_limit_action=2  max_working_current=1 A  power_rating=1 W  enable_faults=0  fault_action=1  lambdaPercent=50  k_faulted=0.9999  turnsShort=0  openCct=0  groundShort=0  groundShortG=0 1/Ohm  tau_fault=1e-3 s  enable_temporal_fault=0  t_fault=1 s  enable_behavioral_fault=0  max_permissible_voltage=100 V  n_fail_on_voltage=1  max_permissible_current=1 A  t_fail_on_current=1 s  i_L_specify=off  i_L_priority=High  i_L=0 A  i_L_nominal_specify=off  i_L_nominal_unit=A  i_L_nominal_value=1
  R : fl_lib/Electrical/Electrical Elements/Resistor  R=4.116 Ohm  i_specify=off  i_priority=None  i=0 A  i_nominal_specify=off  i_nominal_unit=A  i_nominal_value=1  v_specify=off  v_priority=None  v=0 V  v_nominal_specify=off  v_nominal_unit=V  v_nominal_value=1
  Conn1 : PMIOPort  Side=Left
  Conn2 : PMIOPort  Port=2  Side=Right
  Conn3 : PMIOPort  Port=3  Side=Right
  connections:
  R/RConn1 -- L/LConn1
  C/RConn1 -- Conn3/RConn1
  R/LConn1 -- Conn1/RConn1
  C/LConn1 -- L/RConn1 -- Conn2/RConn1

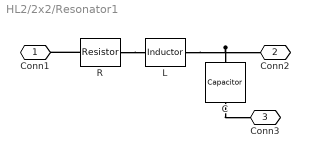
== system HL2/2x2/Resonator1 ==
  C : fl_lib/Electrical/Electrical Elements/Capacitor  c=7.0832e-07 F  r=0 Ohm  g=0 1/Ohm  i_specify=off  i_priority=None  i=0 A  i_nominal_specify=off  i_nominal_unit=A  i_nominal_value=1  v_specify=off  v_priority=None  v=0 V  v_nominal_specify=off  v_nominal_unit=V  v_nominal_value=1  vc_specify=off  vc_priority=High  vc=0 V  vc_nominal_specify=off  vc_nominal_unit=V  vc_nominal_value=1
  L : ee_lib/Passive/Inductor  l=0.10005 H  L_tol=0  enable_L_tol=0  tol_distribution=1  nSigma=4  r=0 Ohm  g=0 1/Ohm  enable_operating_limits=0  operating_limit_action=2  max_working_current=1 A  power_rating=1 W  enable_faults=0  fault_action=1  lambdaPercent=50  k_faulted=0.9999  turnsShort=0  openCct=0  groundShort=0  groundShortG=0 1/Ohm  tau_fault=1e-3 s  enable_temporal_fault=0  t_fault=1 s  enable_behavioral_fault=0  max_permissible_voltage=100 V  n_fail_on_voltage=1  max_permissible_current=1 A  t_fail_on_current=1 s  i_L_specify=off  i_L_priority=High  i_L=0 A  i_L_nominal_specify=off  i_L_nominal_unit=A  i_L_nominal_value=1
  R : fl_lib/Electrical/Electrical Elements/Resistor  R=4.116 Ohm  i_specify=off  i_priority=None  i=0 A  i_nominal_specify=off  i_nominal_unit=A  i_nominal_value=1  v_specify=off  v_priority=None  v=0 V  v_nominal_specify=off  v_nominal_unit=V  v_nominal_value=1
  Conn1 : PMIOPort  Side=Left
  Conn2 : PMIOPort  Port=2  Side=Right
  Conn3 : PMIOPort  Port=3  Side=Right
  connections:
  R/RConn1 -- L/LConn1
  C/RConn1 -- Conn3/RConn1
  R/LConn1 -- Conn1/RConn1
  C/LConn1 -- L/RConn1 -- Conn2/RConn1

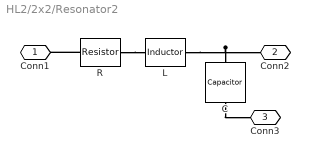
== system HL2/2x2/Resonator2 ==
  C : fl_lib/Electrical/Electrical Elements/Capacitor  c=7.0832e-07 F  r=0 Ohm  g=0 1/Ohm  i_specify=off  i_priority=None  i=0 A  i_nominal_specify=off  i_nominal_unit=A  i_nominal_value=1  v_specify=off  v_priority=None  v=0 V  v_nominal_specify=off  v_nominal_unit=V  v_nominal_value=1  vc_specify=off  vc_priority=High  vc=0 V  vc_nominal_specify=off  vc_nominal_unit=V  vc_nominal_value=1
  L : ee_lib/Passive/Inductor  l=0.10005 H  L_tol=0  enable_L_tol=0  tol_distribution=1  nSigma=4  r=0 Ohm  g=0 1/Ohm  enable_operating_limits=0  operating_limit_action=2  max_working_current=1 A  power_rating=1 W  enable_faults=0  fault_action=1  lambdaPercent=50  k_faulted=0.9999  turnsShort=0  openCct=0  groundShort=0  groundShortG=0 1/Ohm  tau_fault=1e-3 s  enable_temporal_fault=0  t_fault=1 s  enable_behavioral_fault=0  max_permissible_voltage=100 V  n_fail_on_voltage=1  max_permissible_current=1 A  t_fail_on_current=1 s  i_L_specify=off  i_L_priority=High  i_L=0 A  i_L_nominal_specify=off  i_L_nominal_unit=A  i_L_nominal_value=1
  R : fl_lib/Electrical/Electrical Elements/Resistor  R=4.116 Ohm  i_specify=off  i_priority=None  i=0 A  i_nominal_specify=off  i_nominal_unit=A  i_nominal_value=1  v_specify=off  v_priority=None  v=0 V  v_nominal_specify=off  v_nominal_unit=V  v_nominal_value=1
  Conn1 : PMIOPort  Side=Left
  Conn2 : PMIOPort  Port=2  Side=Right
  Conn3 : PMIOPort  Port=3  Side=Right
  connections:
  R/RConn1 -- L/LConn1
  C/RConn1 -- Conn3/RConn1
  R/LConn1 -- Conn1/RConn1
  C/LConn1 -- L/RConn1 -- Conn2/RConn1

== system HL2/2x2/Resonator3 ==
  C : fl_lib/Electrical/Electrical Elements/Capacitor  c=7.0832e-07 F  r=0 Ohm  g=0 1/Ohm  i_specify=off  i_priority=None  i=0 A  i_nominal_specify=off  i_nominal_unit=A  i_nominal_value=1  v_specify=off  v_priority=None  v=0 V  v_nominal_specify=off  v_nominal_unit=V  v_nominal_value=1  vc_specify=off  vc_priority=High  vc=0 V  vc_nominal_specify=off  vc_nominal_unit=V  vc_nominal_value=1
  L : ee_lib/Passive/Inductor  l=0.10005 H  L_tol=0  enable_L_tol=0  tol_distribution=1  nSigma=4  r=0 Ohm  g=0 1/Ohm  enable_operating_limits=0  operating_limit_action=2  max_working_current=1 A  power_rating=1 W  enable_faults=0  fault_action=1  lambdaPercent=50  k_faulted=0.9999  turnsShort=0  openCct=0  groundShort=0  groundShortG=0 1/Ohm  tau_fault=1e-3 s  enable_temporal_fault=0  t_fault=1 s  enable_behavioral_fault=0  max_permissible_voltage=100 V  n_fail_on_voltage=1  max_permissible_current=1 A  t_fail_on_current=1 s  i_L_specify=off  i_L_priority=High  i_L=0 A  i_L_nominal_specify=off  i_L_nominal_unit=A  i_L_nominal_value=1
  R : fl_lib/Electrical/Electrical Elements/Resistor  R=4.116 Ohm  i_specify=off  i_priority=None  i=0 A  i_nominal_specify=off  i_nominal_unit=A  i_nominal_value=1  v_specify=off  v_priority=None  v=0 V  v_nominal_specify=off  v_nominal_unit=V  v_nominal_value=1
  Conn1 : PMIOPort  Side=Left
  Conn2 : PMIOPort  Port=2  Side=Right
  Conn3 : PMIOPort  Port=3  Side=Right
  connections:
  R/RConn1 -- L/LConn1
  C/RConn1 -- Conn3/RConn1
  R/LConn1 -- Conn1/RConn1
  C/LConn1 -- L/RConn1 -- Conn2/RConn1

== system HL2/2x2/Resonator4 ==
  C : fl_lib/Electrical/Electrical Elements/Capacitor  c=7.0832e-07 F  r=0 Ohm  g=0 1/Ohm  i_specify=off  i_priority=None  i=0 A  i_nominal_specify=off  i_nominal_unit=A  i_nominal_value=1  v_specify=off  v_priority=None  v=0 V  v_nominal_specify=off  v_nominal_unit=V  v_nominal_value=1  vc_specify=off  vc_priority=High  vc=0 V  vc_nominal_specify=off  vc_nominal_unit=V  vc_nominal_value=1
  L : ee_lib/Passive/Inductor  l=0.10005 H  L_tol=0  enable_L_tol=0  tol_distribution=1  nSigma=4  r=0 Ohm  g=0 1/Ohm  enable_operating_limits=0  operating_limit_action=2  max_working_current=1 A  power_rating=1 W  enable_faults=0  fault_action=1  lambdaPercent=50  k_faulted=0.9999  turnsShort=0  openCct=0  groundShort=0  groundShortG=0 1/Ohm  tau_fault=1e-3 s  enable_temporal_fault=0  t_fault=1 s  enable_behavioral_fault=0  max_permissible_voltage=100 V  n_fail_on_voltage=1  max_permissible_current=1 A  t_fail_on_current=1 s  i_L_specify=off  i_L_priority=High  i_L=0 A  i_L_nominal_specify=off  i_L_nominal_unit=A  i_L_nominal_value=1
  R : fl_lib/Electrical/Electrical Elements/Resistor  R=4.116 Ohm  i_specify=off  i_priority=None  i=0 A  i_nominal_specify=off  i_nominal_unit=A  i_nominal_value=1  v_specify=off  v_priority=None  v=0 V  v_nominal_specify=off  v_nominal_unit=V  v_nominal_value=1
  Conn1 : PMIOPort  Side=Left
  Conn2 : PMIOPort  Port=2  Side=Right
  Conn3 : PMIOPort  Port=3  Side=Right
  connections:
  R/RConn1 -- L/LConn1
  C/RConn1 -- Conn3/RConn1
  R/LConn1 -- Conn1/RConn1
  C/LConn1 -- L/RConn1 -- Conn2/RConn1

== system HL2/2x2/Resonator5 ==
  C : fl_lib/Electrical/Electrical Elements/Capacitor  c=7.0832e-07 F  r=0 Ohm  g=0 1/Ohm  i_specify=off  i_priority=None  i=0 A  i_nominal_specify=off  i_nominal_unit=A  i_nominal_value=1  v_specify=off  v_priority=None  v=0 V  v_nominal_specify=off  v_nominal_unit=V  v_nominal_value=1  vc_specify=off  vc_priority=High  vc=0 V  vc_nominal_specify=off  vc_nominal_unit=V  vc_nominal_value=1
  L : ee_lib/Passive/Inductor  l=0.10005 H  L_tol=0  enable_L_tol=0  tol_distribution=1  nSigma=4  r=0 Ohm  g=0 1/Ohm  enable_operating_limits=0  operating_limit_action=2  max_working_current=1 A  power_rating=1 W  enable_faults=0  fault_action=1  lambdaPercent=50  k_faulted=0.9999  turnsShort=0  openCct=0  groundShort=0  groundShortG=0 1/Ohm  tau_fault=1e-3 s  enable_temporal_fault=0  t_fault=1 s  enable_behavioral_fault=0  max_permissible_voltage=100 V  n_fail_on_voltage=1  max_permissible_current=1 A  t_fail_on_current=1 s  i_L_specify=off  i_L_priority=High  i_L=0 A  i_L_nominal_specify=off  i_L_nominal_unit=A  i_L_nominal_value=1
  R : fl_lib/Electrical/Electrical Elements/Resistor  R=4.116 Ohm  i_specify=off  i_priority=None  i=0 A  i_nominal_specify=off  i_nominal_unit=A  i_nominal_value=1  v_specify=off  v_priority=None  v=0 V  v_nominal_specify=off  v_nominal_unit=V  v_nominal_value=1
  Conn1 : PMIOPort  Side=Left
  Conn2 : PMIOPort  Port=2  Side=Right
  Conn3 : PMIOPort  Port=3  Side=Right
  connections:
  R/RConn1 -- L/LConn1
  C/RConn1 -- Conn3/RConn1
  R/LConn1 -- Conn1/RConn1
  C/LConn1 -- L/RConn1 -- Conn2/RConn1

== system HL2/2x2/Resonator6 ==
  C : fl_lib/Electrical/Electrical Elements/Capacitor  c=7.0832e-07 F  r=0 Ohm  g=0 1/Ohm  i_specify=off  i_priority=None  i=0 A  i_nominal_specify=off  i_nominal_unit=A  i_nominal_value=1  v_specify=off  v_priority=None  v=0 V  v_nominal_specify=off  v_nominal_unit=V  v_nominal_value=1  vc_specify=off  vc_priority=High  vc=0 V  vc_nominal_specify=off  vc_nominal_unit=V  vc_nominal_value=1
  L : ee_lib/Passive/Inductor  l=0.10005 H  L_tol=0  enable_L_tol=0  tol_distribution=1  nSigma=4  r=0 Ohm  g=0 1/Ohm  enable_operating_limits=0  operating_limit_action=2  max_working_current=1 A  power_rating=1 W  enable_faults=0  fault_action=1  lambdaPercent=50  k_faulted=0.9999  turnsShort=0  openCct=0  groundShort=0  groundShortG=0 1/Ohm  tau_fault=1e-3 s  enable_temporal_fault=0  t_fault=1 s  enable_behavioral_fault=0  max_permissible_voltage=100 V  n_fail_on_voltage=1  max_permissible_current=1 A  t_fail_on_current=1 s  i_L_specify=off  i_L_priority=High  i_L=0 A  i_L_nominal_specify=off  i_L_nominal_unit=A  i_L_nominal_value=1
  R : fl_lib/Electrical/Electrical Elements/Resistor  R=4.116 Ohm  i_specify=off  i_priority=None  i=0 A  i_nominal_specify=off  i_nominal_unit=A  i_nominal_value=1  v_specify=off  v_priority=None  v=0 V  v_nominal_specify=off  v_nominal_unit=V  v_nominal_value=1
  Conn1 : PMIOPort  Side=Left
  Conn2 : PMIOPort  Port=2  Side=Right
  Conn3 : PMIOPort  Port=3  Side=Right
  connections:
  R/RConn1 -- L/LConn1
  C/RConn1 -- Conn3/RConn1
  R/LConn1 -- Conn1/RConn1
  C/LConn1 -- L/RConn1 -- Conn2/RConn1

== system HL2/2x3/Resonator ==
  C : fl_lib/Electrical/Electrical Elements/Capacitor  c=7.0832e-07 F  r=0 Ohm  g=0 1/Ohm  i_specify=off  i_priority=None  i=0 A  i_nominal_specify=off  i_nominal_unit=A  i_nominal_value=1  v_specify=off  v_priority=None  v=0 V  v_nominal_specify=off  v_nominal_unit=V  v_nominal_value=1  vc_specify=off  vc_priority=High  vc=0 V  vc_nominal_specify=off  vc_nominal_unit=V  vc_nominal_value=1
  L : ee_lib/Passive/Inductor  l=0.10005 H  L_tol=0  enable_L_tol=0  tol_distribution=1  nSigma=4  r=0 Ohm  g=0 1/Ohm  enable_operating_limits=0  operating_limit_action=2  max_working_current=1 A  power_rating=1 W  enable_faults=0  fault_action=1  lambdaPercent=50  k_faulted=0.9999  turnsShort=0  openCct=0  groundShort=0  groundShortG=0 1/Ohm  tau_fault=1e-3 s  enable_temporal_fault=0  t_fault=1 s  enable_behavioral_fault=0  max_permissible_voltage=100 V  n_fail_on_voltage=1  max_permissible_current=1 A  t_fail_on_current=1 s  i_L_specify=off  i_L_priority=High  i_L=0 A  i_L_nominal_specify=off  i_L_nominal_unit=A  i_L_nominal_value=1
  R : fl_lib/Electrical/Electrical Elements/Resistor  R=4.116 Ohm  i_specify=off  i_priority=None  i=0 A  i_nominal_specify=off  i_nominal_unit=A  i_nominal_value=1  v_specify=off  v_priority=None  v=0 V  v_nominal_specify=off  v_nominal_unit=V  v_nominal_value=1
  Conn1 : PMIOPort  Side=Left
  Conn2 : PMIOPort  Port=2  Side=Right
  Conn3 : PMIOPort  Port=3  Side=Right
  connections:
  R/RConn1 -- L/LConn1
  C/RConn1 -- Conn3/RConn1
  R/LConn1 -- Conn1/RConn1
  C/LConn1 -- L/RConn1 -- Conn2/RConn1

== system HL2/2x3/Resonator1 ==
  C : fl_lib/Electrical/Electrical Elements/Capacitor  c=7.0832e-07 F  r=0 Ohm  g=0 1/Ohm  i_specify=off  i_priority=None  i=0 A  i_nominal_specify=off  i_nominal_unit=A  i_nominal_value=1  v_specify=off  v_priority=None  v=0 V  v_nominal_specify=off  v_nominal_unit=V  v_nominal_value=1  vc_specify=off  vc_priority=High  vc=0 V  vc_nominal_specify=off  vc_nominal_unit=V  vc_nominal_value=1
  L : ee_lib/Passive/Inductor  l=0.10005 H  L_tol=0  enable_L_tol=0  tol_distribution=1  nSigma=4  r=0 Ohm  g=0 1/Ohm  enable_operating_limits=0  operating_limit_action=2  max_working_current=1 A  power_rating=1 W  enable_faults=0  fault_action=1  lambdaPercent=50  k_faulted=0.9999  turnsShort=0  openCct=0  groundShort=0  groundShortG=0 1/Ohm  tau_fault=1e-3 s  enable_temporal_fault=0  t_fault=1 s  enable_behavioral_fault=0  max_permissible_voltage=100 V  n_fail_on_voltage=1  max_permissible_current=1 A  t_fail_on_current=1 s  i_L_specify=off  i_L_priority=High  i_L=0 A  i_L_nominal_specify=off  i_L_nominal_unit=A  i_L_nominal_value=1
  R : fl_lib/Electrical/Electrical Elements/Resistor  R=4.116 Ohm  i_specify=off  i_priority=None  i=0 A  i_nominal_specify=off  i_nominal_unit=A  i_nominal_value=1  v_specify=off  v_priority=None  v=0 V  v_nominal_specify=off  v_nominal_unit=V  v_nominal_value=1
  Conn1 : PMIOPort  Side=Left
  Conn2 : PMIOPort  Port=2  Side=Right
  Conn3 : PMIOPort  Port=3  Side=Right
  connections:
  R/RConn1 -- L/LConn1
  C/RConn1 -- Conn3/RConn1
  R/LConn1 -- Conn1/RConn1
  C/LConn1 -- L/RConn1 -- Conn2/RConn1

== system HL2/2x3/Resonator10 ==
  C : fl_lib/Electrical/Electrical Elements/Capacitor  c=7.0832e-07 F  r=0 Ohm  g=0 1/Ohm  i_specify=off  i_priority=None  i=0 A  i_nominal_specify=off  i_nominal_unit=A  i_nominal_value=1  v_specify=off  v_priority=None  v=0 V  v_nominal_specify=off  v_nominal_unit=V  v_nominal_value=1  vc_specify=off  vc_priority=High  vc=0 V  vc_nominal_specify=off  vc_nominal_unit=V  vc_nominal_value=1
  L : ee_lib/Passive/Inductor  l=0.10005 H  L_tol=0  enable_L_tol=0  tol_distribution=1  nSigma=4  r=0 Ohm  g=0 1/Ohm  enable_operating_limits=0  operating_limit_action=2  max_working_current=1 A  power_rating=1 W  enable_faults=0  fault_action=1  lambdaPercent=50  k_faulted=0.9999  turnsShort=0  openCct=0  groundShort=0  groundShortG=0 1/Ohm  tau_fault=1e-3 s  enable_temporal_fault=0  t_fault=1 s  enable_behavioral_fault=0  max_permissible_voltage=100 V  n_fail_on_voltage=1  max_permissible_current=1 A  t_fail_on_current=1 s  i_L_specify=off  i_L_priority=High  i_L=0 A  i_L_nominal_specify=off  i_L_nominal_unit=A  i_L_nominal_value=1
  R : fl_lib/Electrical/Electrical Elements/Resistor  R=4.116 Ohm  i_specify=off  i_priority=None  i=0 A  i_nominal_specify=off  i_nominal_unit=A  i_nominal_value=1  v_specify=off  v_priority=None  v=0 V  v_nominal_specify=off  v_nominal_unit=V  v_nominal_value=1
  Conn1 : PMIOPort  Side=Left
  Conn2 : PMIOPort  Port=2  Side=Right
  Conn3 : PMIOPort  Port=3  Side=Right
  connections:
  R/RConn1 -- L/LConn1
  C/RConn1 -- Conn3/RConn1
  R/LConn1 -- Conn1/RConn1
  C/LConn1 -- L/RConn1 -- Conn2/RConn1

== system HL2/2x3/Resonator11 ==
  C : fl_lib/Electrical/Electrical Elements/Capacitor  c=7.0832e-07 F  r=0 Ohm  g=0 1/Ohm  i_specify=off  i_priority=None  i=0 A  i_nominal_specify=off  i_nominal_unit=A  i_nominal_value=1  v_specify=off  v_priority=None  v=0 V  v_nominal_specify=off  v_nominal_unit=V  v_nominal_value=1  vc_specify=off  vc_priority=High  vc=0 V  vc_nominal_specify=off  vc_nominal_unit=V  vc_nominal_value=1
  L : ee_lib/Passive/Inductor  l=0.10005 H  L_tol=0  enable_L_tol=0  tol_distribution=1  nSigma=4  r=0 Ohm  g=0 1/Ohm  enable_operating_limits=0  operating_limit_action=2  max_working_current=1 A  power_rating=1 W  enable_faults=0  fault_action=1  lambdaPercent=50  k_faulted=0.9999  turnsShort=0  openCct=0  groundShort=0  groundShortG=0 1/Ohm  tau_fault=1e-3 s  enable_temporal_fault=0  t_fault=1 s  enable_behavioral_fault=0  max_permissible_voltage=100 V  n_fail_on_voltage=1  max_permissible_current=1 A  t_fail_on_current=1 s  i_L_specify=off  i_L_priority=High  i_L=0 A  i_L_nominal_specify=off  i_L_nominal_unit=A  i_L_nominal_value=1
  R : fl_lib/Electrical/Electrical Elements/Resistor  R=4.116 Ohm  i_specify=off  i_priority=None  i=0 A  i_nominal_specify=off  i_nominal_unit=A  i_nominal_value=1  v_specify=off  v_priority=None  v=0 V  v_nominal_specify=off  v_nominal_unit=V  v_nominal_value=1
  Conn1 : PMIOPort  Side=Left
  Conn2 : PMIOPort  Port=2  Side=Right
  Conn3 : PMIOPort  Port=3  Side=Right
  connections:
  R/RConn1 -- L/LConn1
  C/RConn1 -- Conn3/RConn1
  R/LConn1 -- Conn1/RConn1
  C/LConn1 -- L/RConn1 -- Conn2/RConn1
